simulink model "tentando_debugar_3"  (R2012b)
settings: Solver=ode45  StartTime=0.0  StopTime=1  RelTol=1e-3
undefined symbols (not defined in the file): DF, DiscIntNeverNeededParam, J, Kd, Ke, KE, Kt, KT, L, P, R, Ts
libraries: simulink x4
settings Model: Creator=Juliano  LastModifiedBy=Juliano

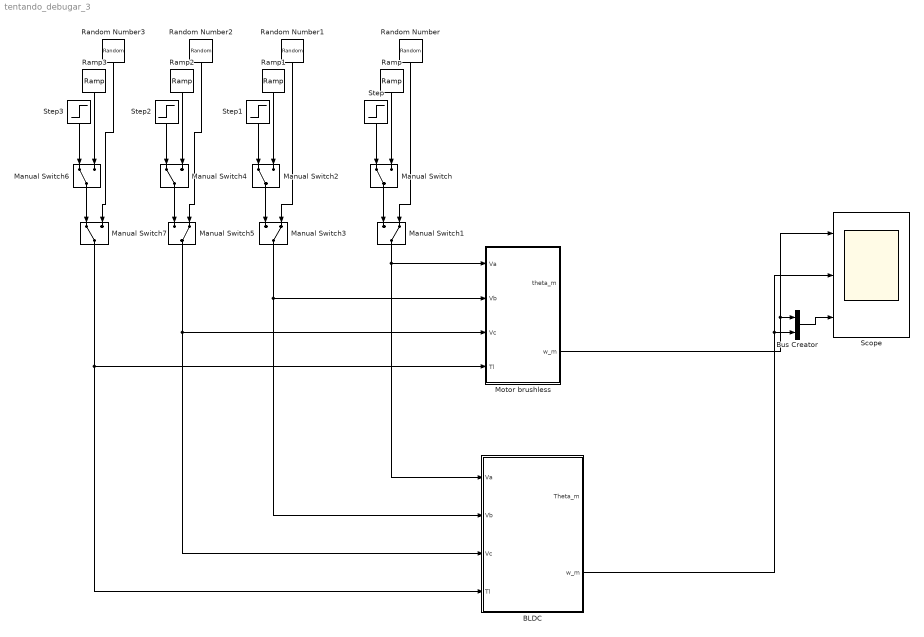
== system tentando_debugar_3 ==
  BLDC : Subsystem
  Bus Creator : BusCreator  Inputs=2
  Manual Switch{,2,4,6..7} (5 alike) : ManualSwitch
  Manual Switch1 : ManualSwitch  CurrentSetting=0
  Manual Switch3 : ManualSwitch  CurrentSetting=0
  Manual Switch5 : ManualSwitch  CurrentSetting=0
  Motor brushless : Subsystem
  Ramp{,1..3} (4 alike) : simulink/Sources/Ramp  slope=2*pi  start=0  X0=0
  Random Number : RandomNumber  SampleTime=0.1
  Random Number1 : RandomNumber  Seed=1  SampleTime=0.1
  Random Number2 : RandomNumber  Seed=2  SampleTime=0.1
  Random Number3 : RandomNumber  Seed=3  SampleTime=0.1
  Scope : Scope  NumInputPorts=3
      settings: TimeRange=0.5  YMin=-60~-60~-60  YMax=70~70~70
  Step : Step  Time=0  After=12  SampleTime=0
  Step1 : Step  Time=0  After=12  SampleTime=0
  Step2 : Step  Time=0  After=12  SampleTime=0
  Step3 : Step  Time=0  After=0  SampleTime=0
  wires:
  Step/1 -> Manual Switch/1
  Ramp/1 -> Manual Switch/2
  Random Number/1 -> Manual Switch1/2
  Manual Switch/1 -> Manual Switch1/1
  Manual Switch1/1 -> BLDC/1(Va), Motor brushless/1(Va)
  Step1/1 -> Manual Switch2/1
  Ramp1/1 -> Manual Switch2/2
  Random Number1/1 -> Manual Switch3/2
  Manual Switch2/1 -> Manual Switch3/1
  Step2/1 -> Manual Switch4/1
  Ramp2/1 -> Manual Switch4/2
  Random Number2/1 -> Manual Switch5/2
  Manual Switch4/1 -> Manual Switch5/1
  Step3/1 -> Manual Switch6/1
  Ramp3/1 -> Manual Switch6/2
  Random Number3/1 -> Manual Switch7/2
  Manual Switch6/1 -> Manual Switch7/1
  Manual Switch3/1 -> BLDC/2(Vb), Motor brushless/2(Vb)
  Manual Switch5/1 -> BLDC/3(Vc), Motor brushless/3(Vc)
  Manual Switch7/1 -> BLDC/4(Tl), Motor brushless/4(Tl)
  Motor brushless/2(w_m) -> Scope/1, Bus Creator/1
  BLDC/2(w_m) -> Scope/2, Bus Creator/2
  Bus Creator/1 -> Scope/3

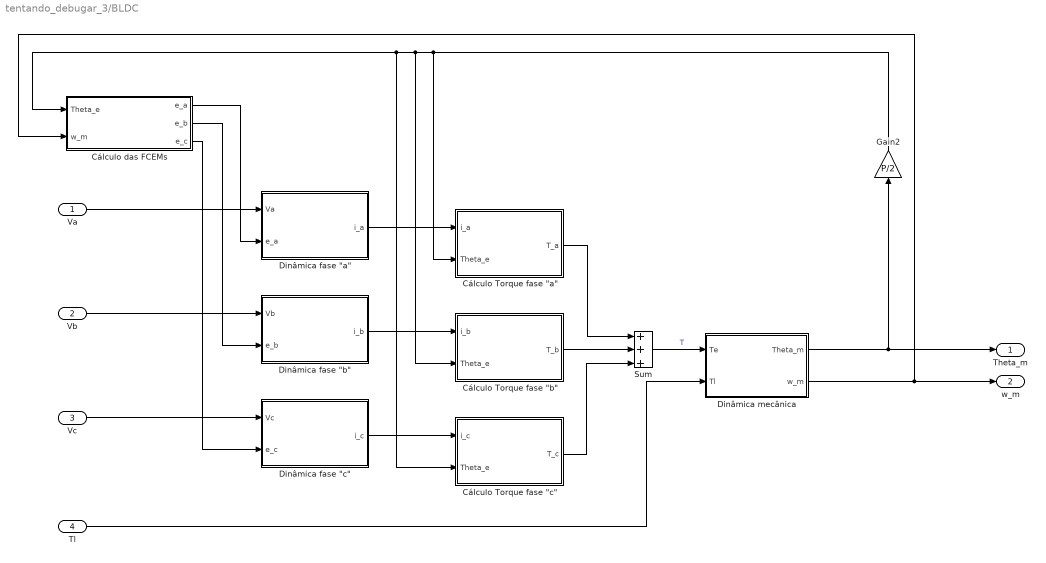
== system tentando_debugar_3/BLDC ==
  Va : Inport
  Vb : Inport  Port=2
  Vc : Inport  Port=3
  Tl : Inport  Port=4
  "Cálculo Torque fase \"a\"" : Subsystem
  "Cálculo Torque fase \"b\"" : Subsystem
  "Cálculo Torque fase \"c\"" : Subsystem
  Cálculo das FCEMs : Subsystem
  "Dinâmica fase \"a\"" : Subsystem
  "Dinâmica fase \"b\"" : Subsystem
  "Dinâmica fase \"c\"" : Subsystem
  "Dinâmica mecânica " : Subsystem
  Gain2 : Gain  Gain=P/2
  Sum : Sum  Inputs=+++
  Theta_m : Outport
  w_m : Outport  Port=2
  wires:
  Gain2/1 -> "Cálculo Torque fase \"b\""/2(Theta_e), Cálculo das FCEMs/1(Theta_e), "Cálculo Torque fase \"c\""/2(Theta_e), "Cálculo Torque fase \"a\""/2(Theta_e)
  Tl/1 -> "Dinâmica mecânica "/2(Tl)
  "Dinâmica mecânica "/2(w_m) -> w_m/1, Cálculo das FCEMs/2(w_m)
  "Dinâmica mecânica "/1(Theta_m) -> Gain2/1, Theta_m/1
  Sum/1 -> "Dinâmica mecânica "/1(Te)  "T"
  "Cálculo Torque fase \"c\""/1(T_c) -> Sum/3
  "Cálculo Torque fase \"b\""/1(T_b) -> Sum/2
  "Cálculo Torque fase \"a\""/1(T_a) -> Sum/1
  "Dinâmica fase \"c\""/1(i_c) -> "Cálculo Torque fase \"c\""/1(i_c)
  "Dinâmica fase \"b\""/1(i_b) -> "Cálculo Torque fase \"b\""/1(i_b)
  "Dinâmica fase \"a\""/1(i_a) -> "Cálculo Torque fase \"a\""/1(i_a)
  Vc/1 -> "Dinâmica fase \"c\""/1(Vc)
  Vb/1 -> "Dinâmica fase \"b\""/1(Vb)
  Va/1 -> "Dinâmica fase \"a\""/1(Va)
  Cálculo das FCEMs/3(e_c) -> "Dinâmica fase \"c\""/2(e_c)
  Cálculo das FCEMs/2(e_b) -> "Dinâmica fase \"b\""/2(e_b)
  Cálculo das FCEMs/1(e_a) -> "Dinâmica fase \"a\""/2(e_a)

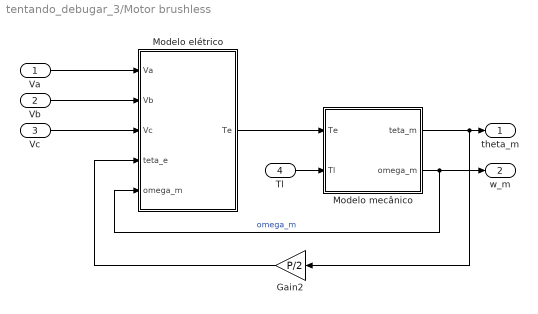
== system tentando_debugar_3/Motor brushless ==
  Va : Inport
  Vb : Inport  Port=2
  Vc : Inport  Port=3
  Tl : Inport  Port=4
  Gain2 : Gain  Gain=P/2
  Modelo elétrico : Subsystem
  Modelo mecânico : Subsystem
  theta_m : Outport
  w_m : Outport  Port=2
  wires:
  Modelo elétrico/1(Te) -> Modelo mecânico/1(Te)
  Modelo mecânico/1(teta_m) -> theta_m/1, Gain2/1
  Va/1 -> Modelo elétrico/1(Va)
  Vb/1 -> Modelo elétrico/2(Vb)
  Vc/1 -> Modelo elétrico/3(Vc)
  Tl/1 -> Modelo mecânico/2(Tl)
  Modelo mecânico/2(omega_m) -> w_m/1, Modelo elétrico/5(omega_m)  "omega_m"
  Gain2/1 -> Modelo elétrico/4(teta_e)

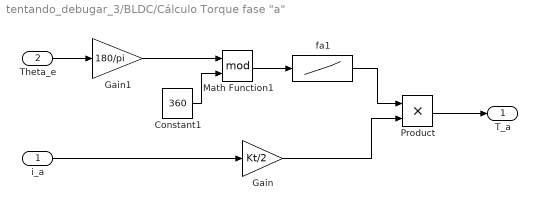
== system tentando_debugar_3/BLDC/Cálculo Torque fase "a" ==
  i_a : Inport
  Theta_e : Inport  Port=2
  Constant1 : Constant  Value=360
  Gain : Gain  Gain=Kt/2
  Gain1 : Gain  Gain=180/pi
  Math Function1 : Math  Operator=mod  SaturateOnIntegerOverflow=on
  Product : Product  RndMeth=Zero
  fa1 : Lookup  InputValues=[0 30 60 90 120 150 180 210 240 270 300 330 360]  Table=[ 1 1 1 0 -1 -1 -1 -1 -1 0 1 1 1]
  T_a : Outport
  wires:
  Constant1/1 -> Math Function1/2
  Gain1/1 -> Math Function1/1
  Product/1 -> T_a/1
  fa1/1 -> Product/1
  Theta_e/1 -> Gain1/1
  Math Function1/1 -> fa1/1
  Gain/1 -> Product/2
  i_a/1 -> Gain/1

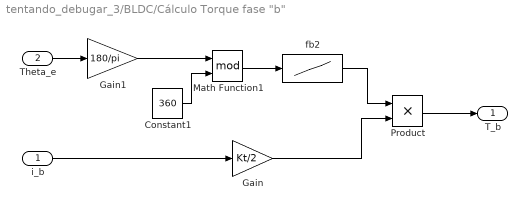
== system tentando_debugar_3/BLDC/Cálculo Torque fase "b" ==
  i_b : Inport
  Theta_e : Inport  Port=2
  Constant1 : Constant  Value=360
  Gain : Gain  Gain=Kt/2
  Gain1 : Gain  Gain=180/pi
  Math Function1 : Math  Operator=mod  SaturateOnIntegerOverflow=on
  Product : Product  RndMeth=Zero
  fb2 : Lookup  InputValues=[0 30 60 90 120 150 180 210 240 270 300 330 360]  Table=[-1 0 1 1 1 1 1 0 -1 -1 -1 -1 -1]
  T_b : Outport
  wires:
  Constant1/1 -> Math Function1/2
  Gain1/1 -> Math Function1/1
  i_b/1 -> Gain/1
  Gain/1 -> Product/2
  Math Function1/1 -> fb2/1
  Theta_e/1 -> Gain1/1
  fb2/1 -> Product/1
  Product/1 -> T_b/1

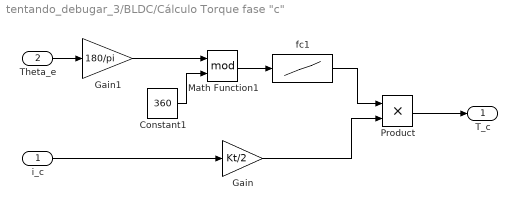
== system tentando_debugar_3/BLDC/Cálculo Torque fase "c" ==
  i_c : Inport
  Theta_e : Inport  Port=2
  Constant1 : Constant  Value=360
  Gain : Gain  Gain=Kt/2
  Gain1 : Gain  Gain=180/pi
  Math Function1 : Math  Operator=mod  SaturateOnIntegerOverflow=on
  Product : Product  RndMeth=Zero
  fc1 : Lookup  InputValues=[0 30 60 90 120 150 180 210 240 270 300 330 360]  Table=[-1 -1 -1 -1 -1 0 1 1 1 1 1 0 -1]
  T_c : Outport
  wires:
  Constant1/1 -> Math Function1/2
  Gain1/1 -> Math Function1/1
  Product/1 -> T_c/1
  fc1/1 -> Product/1
  Theta_e/1 -> Gain1/1
  Math Function1/1 -> fc1/1
  Gain/1 -> Product/2
  i_c/1 -> Gain/1

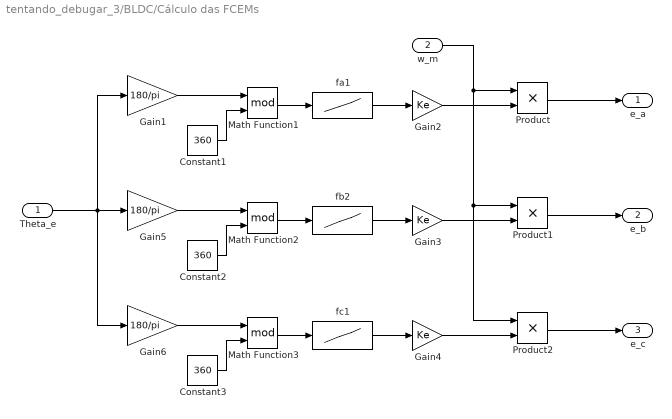
== system tentando_debugar_3/BLDC/Cálculo das FCEMs ==
  Theta_e : Inport
  w_m : Inport  Port=2
  Constant1 : Constant  Value=360
  Constant2 : Constant  Value=360
  Constant3 : Constant  Value=360
  Gain1 : Gain  Gain=180/pi
  Gain2 : Gain  Gain=Ke
  Gain3 : Gain  Gain=Ke
  Gain4 : Gain  Gain=Ke
  Gain5 : Gain  Gain=180/pi
  Gain6 : Gain  Gain=180/pi
  Math Function1 : Math  Operator=mod  SaturateOnIntegerOverflow=on
  Math Function2 : Math  Operator=mod  SaturateOnIntegerOverflow=on
  Math Function3 : Math  Operator=mod  SaturateOnIntegerOverflow=on
  Product : Product  RndMeth=Zero
  Product1 : Product  RndMeth=Zero
  Product2 : Product  RndMeth=Zero
  fa1 : Lookup  InputValues=[0 30 60 90 120 150 180 210 240 270 300 330 360]  Table=[ 1 1 1 0 -1 -1 -1 -1 -1 0 1 1 1]
  fb2 : Lookup  InputValues=[0 30 60 90 120 150 180 210 240 270 300 330 360]  Table=[-1 0 1 1 1 1 1 0 -1 -1 -1 -1 -1]
  fc1 : Lookup  InputValues=[0 30 60 90 120 150 180 210 240 270 300 330 360]  Table=[-1 -1 -1 -1 -1 0 1 1 1 1 1 0 -1]
  e_a : Outport
  e_b : Outport  Port=2
  e_c : Outport  Port=3
  wires:
  Constant3/1 -> Math Function3/2
  Constant2/1 -> Math Function2/2
  Constant1/1 -> Math Function1/2
  Product/1 -> e_a/1
  Product1/1 -> e_b/1
  Theta_e/1 -> Gain5/1, Gain1/1, Gain6/1
  Product2/1 -> e_c/1
  Gain2/1 -> Product/2
  w_m/1 -> Product/1, Product1/1, Product2/1
  Gain3/1 -> Product1/2
  Gain4/1 -> Product2/2
  Gain1/1 -> Math Function1/1
  Gain5/1 -> Math Function2/1
  Gain6/1 -> Math Function3/1
  Math Function1/1 -> fa1/1
  fa1/1 -> Gain2/1
  Math Function2/1 -> fb2/1
  fb2/1 -> Gain3/1
  Math Function3/1 -> fc1/1
  fc1/1 -> Gain4/1

== system tentando_debugar_3/BLDC/Dinâmica fase "a" ==
  note: Gain
  Va : Inport
  e_a : Inport  Port=2
  " " : Gain  Gain=1/L
  Gain : Gain  Gain=R
  Integrator : Integrator
  Sum : Sum  Inputs=+--
  i_a : Outport
  wires:
  e_a/1 -> Sum/2
  Gain/1 -> Sum/3
  " "/1 -> Integrator/1
  Sum/1 -> " "/1
  Va/1 -> Sum/1
  Integrator/1 -> Gain/1, i_a/1

== system tentando_debugar_3/BLDC/Dinâmica fase "b" ==
  note: Gain
  Vb : Inport
  e_b : Inport  Port=2
  " " : Gain  Gain=1/L
  Gain : Gain  Gain=R
  Integrator : Integrator
  Sum : Sum  Inputs=+--
  i_b : Outport
  wires:
  Integrator/1 -> i_b/1, Gain/1
  Vb/1 -> Sum/1
  Sum/1 -> " "/1
  " "/1 -> Integrator/1
  Gain/1 -> Sum/3
  e_b/1 -> Sum/2

== system tentando_debugar_3/BLDC/Dinâmica fase "c" ==
  note: Gain
  Vc : Inport
  e_c : Inport  Port=2
  " " : Gain  Gain=1/L
  Gain : Gain  Gain=R
  Integrator : Integrator
  Sum : Sum  Inputs=+--
  i_c : Outport
  wires:
  e_c/1 -> Sum/2
  Gain/1 -> Sum/3
  " "/1 -> Integrator/1
  Sum/1 -> " "/1
  Vc/1 -> Sum/1
  Integrator/1 -> Gain/1, i_c/1

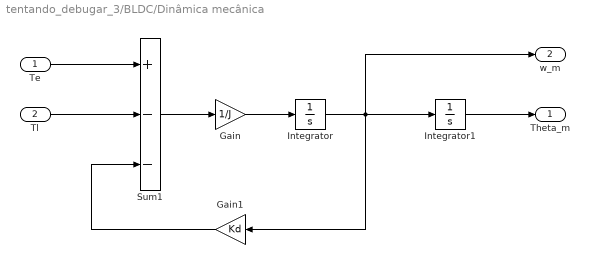
== system tentando_debugar_3/BLDC/Dinâmica mecânica  ==
  Te : Inport
  Tl : Inport  Port=2
  Gain : Gain  Gain=1/J
  Gain1 : Gain  Gain=Kd
  Integrator : Integrator
  Integrator1 : Integrator
  Sum1 : Sum  Inputs=+--
  Theta_m : Outport
  w_m : Outport  Port=2
  wires:
  Integrator1/1 -> Theta_m/1
  Tl/1 -> Sum1/2
  Gain1/1 -> Sum1/3
  Te/1 -> Sum1/1
  Integrator/1 -> Gain1/1, Integrator1/1, w_m/1
  Gain/1 -> Integrator/1
  Sum1/1 -> Gain/1

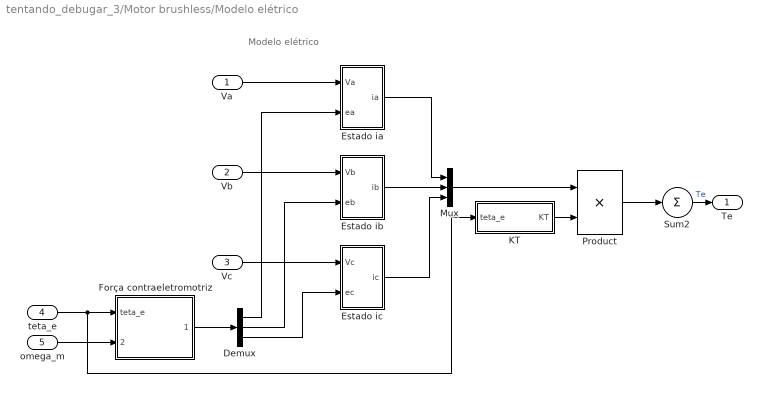
== system tentando_debugar_3/Motor brushless/Modelo elétrico ==
  note: Modelo elétrico
  Va : Inport
  Vb : Inport  Port=2
  Vc : Inport  Port=3
  teta_e : Inport  Port=4
  omega_m : Inport  Port=5
  Demux : Demux  Outputs=3
  Estado ia : Subsystem
  Estado ib : Subsystem
  Estado ic : Subsystem
  Força contraeletromotriz : Subsystem
  KT : Subsystem
  Mux : Mux  Inputs=3
  Product : Product  SaturateOnIntegerOverflow=on  OutDataTypeStr=Inherit: Same as first input
  Sum2 : Sum  Inputs=+  SaturateOnIntegerOverflow=on
  Te : Outport
  wires:
  Estado ic/1(ic) -> Mux/3
  Estado ib/1(ib) -> Mux/2
  Vb/1 -> Estado ib/1(Vb)
  Estado ia/1(ia) -> Mux/1
  Va/1 -> Estado ia/1(Va)
  teta_e/1 -> KT/1(teta_e), Força contraeletromotriz/1(teta_e)
  omega_m/1 -> Força contraeletromotriz/2(omega_e)
  Força contraeletromotriz/1(Fcem abc) -> Demux/1
  Demux/2 -> Estado ib/2(eb)
  Demux/1 -> Estado ia/2(ea)
  KT/1(KT) -> Product/2
  Product/1 -> Sum2/1
  Sum2/1 -> Te/1  "Te"
  Demux/3 -> Estado ic/2(ec)
  Vc/1 -> Estado ic/1(Vc)
  Mux/1 -> Product/1

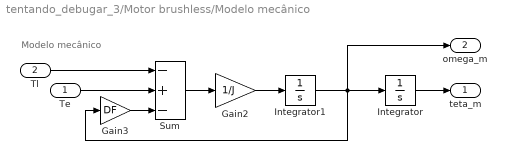
== system tentando_debugar_3/Motor brushless/Modelo mecânico ==
  note: Modelo mecânico
  Te : Inport
  Tl : Inport  Port=2
  Gain2 : Gain  Gain=1/J  SaturateOnIntegerOverflow=on  OutDataTypeStr=Inherit: Same as input  ParamDataTypeStr=Inherit: Same as input
  Gain3 : Gain  Gain=DF  SaturateOnIntegerOverflow=on  OutDataTypeStr=Inherit: Same as input  ParamDataTypeStr=Inherit: Same as input
  Integrator : Integrator
  Integrator1 : Integrator
  Sum : Sum  Inputs=-+-  SaturateOnIntegerOverflow=on  InputSameDT=on  OutDataTypeStr=Inherit: Same as first input
  teta_m : Outport
  omega_m : Outport  Port=2
  wires:
  Integrator1/1 -> Gain3/1, omega_m/1, Integrator/1
  Gain2/1 -> Integrator1/1
  Sum/1 -> Gain2/1
  Tl/1 -> Sum/1
  Gain3/1 -> Sum/3
  Te/1 -> Sum/2
  Integrator/1 -> teta_m/1

== system tentando_debugar_3/Motor brushless/Modelo elétrico/Estado ia ==
  Va : Inport
  ea : Inport  Port=2
  Discrete-Time Integrator : DiscreteIntegrator  SampleTime=Ts  ICPrevOutput=DiscIntNeverNeededParam  ICPrevScaledInput=DiscIntNeverNeededParam
  Fcn : Fcn  Expr=u(1)-(R*u(3))-(u(2))
  Gain : Gain  Gain=1/L
  Mux : Mux  Inputs=3
  ia : Outport
  wires:
  Va/1 -> Mux/1
  ea/1 -> Mux/2
  Mux/1 -> Fcn/1
  Fcn/1 -> Gain/1
  Discrete-Time Integrator/1 -> ia/1, Mux/3  "ia"
  Gain/1 -> Discrete-Time Integrator/1

== system tentando_debugar_3/Motor brushless/Modelo elétrico/Estado ib ==
  Vb : Inport
  eb : Inport  Port=2
  Discrete-Time Integrator : DiscreteIntegrator  SampleTime=Ts  ICPrevOutput=DiscIntNeverNeededParam  ICPrevScaledInput=DiscIntNeverNeededParam
  Fcn : Fcn  Expr=(u(1))-(R*u(3))-(u(2))
  Gain : Gain  Gain=1/L
  Mux : Mux  Inputs=3
  ib : Outport
  wires:
  Vb/1 -> Mux/1
  eb/1 -> Mux/2
  Mux/1 -> Fcn/1
  Fcn/1 -> Gain/1
  Discrete-Time Integrator/1 -> ib/1, Mux/3  "ib"
  Gain/1 -> Discrete-Time Integrator/1

== system tentando_debugar_3/Motor brushless/Modelo elétrico/Estado ic ==
  Vc : Inport
  ec : Inport  Port=2
  Discrete-Time Integrator : DiscreteIntegrator  SampleTime=Ts  ICPrevOutput=DiscIntNeverNeededParam  ICPrevScaledInput=DiscIntNeverNeededParam
  Fcn1 : Fcn  Expr=(u(1))-(R*u(3))-(u(2))
  Gain : Gain  Gain=1/L
  Mux : Mux  Inputs=3
  ic : Outport
  wires:
  Vc/1 -> Mux/1
  ec/1 -> Mux/2
  Mux/1 -> Fcn1/1
  Fcn1/1 -> Gain/1  "ic"
  Discrete-Time Integrator/1 -> ic/1, Mux/3  "ic"
  Gain/1 -> Discrete-Time Integrator/1

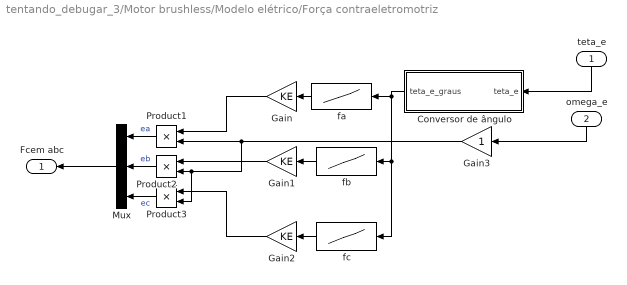
== system tentando_debugar_3/Motor brushless/Modelo elétrico/Força contraeletromotriz ==
  teta_e : Inport
  omega_e : Inport  Port=2
  Conversor de ângulo : Subsystem
  Gain : Gain  Gain=KE
  Gain1 : Gain  Gain=KE
  Gain2 : Gain  Gain=KE
  Gain3 : Gain
  Mux : Mux  Inputs=3
  Product1 : Product  SaturateOnIntegerOverflow=on  OutDataTypeStr=Inherit: Same as first input
  Product2 : Product  SaturateOnIntegerOverflow=on  OutDataTypeStr=Inherit: Same as first input
  Product3 : Product  SaturateOnIntegerOverflow=on  OutDataTypeStr=Inherit: Same as first input
  fa : Lookup  InputValues=[-180 -150 -120 -90 -60 -30 0 30 60 90 120 150 180]  Table=[-1 -1 -1 0 1 1 1 1 1 0 -1 -1 -1]
  fb : Lookup  InputValues=[-180 -150 -120 -90 -60 -30 0 30 60 90 120 150 180]  Table="[1 0 -1 -1 -1 -1  -1 0 1 1 1 1 1]"
  fc : Lookup  InputValues=[-180 -150 -120 -90 -60 -30 0 30 60 90 120 150 180]  Table=[1 1 1 1 1 0 -1 -1 -1 -1 -1 0 1]
  Fcem abc : Outport
  wires:
  fa/1 -> Gain/1
  fb/1 -> Gain1/1
  fc/1 -> Gain2/1
  teta_e/1 -> Conversor de ângulo/1(teta_e)
  Mux/1 -> Fcem abc/1
  Conversor de ângulo/1(teta_e_graus) -> fa/1, fc/1, fb/1
  Product1/1 -> Mux/1  "ea"
  Product2/1 -> Mux/2  "eb"
  Product3/1 -> Mux/3  "ec"
  Gain/1 -> Product1/1
  Gain1/1 -> Product2/1
  Gain2/1 -> Product3/1
  omega_e/1 -> Gain3/1
  Gain3/1 -> Product1/2, Product2/2, Product3/2

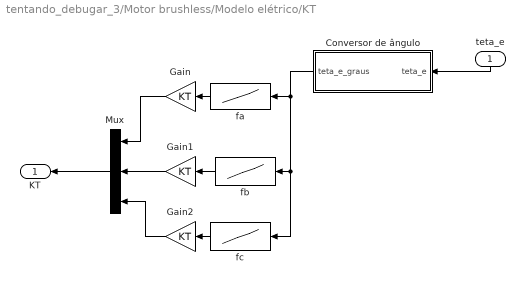
== system tentando_debugar_3/Motor brushless/Modelo elétrico/KT ==
  teta_e : Inport
  Conversor de ângulo : Subsystem
  Gain : Gain  Gain=KT
  Gain1 : Gain  Gain=KT
  Gain2 : Gain  Gain=KT
  Mux : Mux  Inputs=3
  fa : Lookup  InputValues=[-180 -150 -120 -90 -60 -30 0 30 60 90 120 150 180]  Table=[-1 -1 -1 0 1 1 1 1 1 0 -1 -1 -1]
  fb : Lookup  InputValues=[-180 -150 -120 -90 -60 -30 0 30 60 90 120 150 180]  Table="[1 0 -1 -1 -1 -1  -1 0 1 1 1 1 1]"
  fc : Lookup  InputValues=[-180 -150 -120 -90 -60 -30 0 30 60 90 120 150 180]  Table=[1 1 1 1 1 0 -1 -1 -1 -1 -1 0 1]
  KT : Outport
  wires:
  fa/1 -> Gain/1
  fb/1 -> Gain1/1
  fc/1 -> Gain2/1
  teta_e/1 -> Conversor de ângulo/1(teta_e)
  Gain/1 -> Mux/1
  Gain1/1 -> Mux/2
  Gain2/1 -> Mux/3
  Mux/1 -> KT/1
  Conversor de ângulo/1(teta_e_graus) -> fb/1, fc/1, fa/1

== system tentando_debugar_3/Motor brushless/Modelo elétrico/Força contraeletromotriz/Conversor de ângulo ==
  note: Este subsistema converte um ângulo que varia de 0° a infinito
      | para um ângulo variando entre -180° a 180°
  teta_e : Inport
  Trigonometric Function : Trigonometry
  Trigonometric Function1 : Trigonometry  Operator=cos
  Trigonometric Function2 : Trigonometry  Operator=atan2
  rad2graus : Gain  Gain=180/pi  SaturateOnIntegerOverflow=on  OutDataTypeStr=Inherit: Same as input  ParamDataTypeStr=Inherit: Same as input
  teta_e_graus : Outport
  wires:
  teta_e/1 -> Trigonometric Function/1, Trigonometric Function1/1
  Trigonometric Function/1 -> Trigonometric Function2/1
  Trigonometric Function1/1 -> Trigonometric Function2/2
  Trigonometric Function2/1 -> rad2graus/1
  rad2graus/1 -> teta_e_graus/1

== system tentando_debugar_3/Motor brushless/Modelo elétrico/KT/Conversor de ângulo ==
  note: Este subsistema converte um ângulo que varia de 0° a infinito
      | para um ângulo variando entre -180° a 180°
  teta_e : Inport
  Trigonometric Function : Trigonometry
  Trigonometric Function1 : Trigonometry  Operator=cos
  Trigonometric Function2 : Trigonometry  Operator=atan2
  rad2graus : Gain  Gain=180/pi  SaturateOnIntegerOverflow=on  OutDataTypeStr=Inherit: Same as input  ParamDataTypeStr=Inherit: Same as input
  teta_e_graus : Outport
  wires:
  teta_e/1 -> Trigonometric Function/1, Trigonometric Function1/1
  Trigonometric Function/1 -> Trigonometric Function2/1
  Trigonometric Function1/1 -> Trigonometric Function2/2
  Trigonometric Function2/1 -> rad2graus/1
  rad2graus/1 -> teta_e_graus/1
